simulink model "SF103A_MotRefMdl"  (R2013b)
settings: Solver=FixedStepDiscrete  StartTime=0.0  StopTime=2  FixedStep=.002  RelTol=1e-3
values from neighbouring files (symbols this model uses):
  ARCHGLBPRM_2MILLISEC_SEC_F32 = DataDict.Constant    [SF103A_MotRefMdl_DataDict.m]
  ARCHGLBPRM_2OVERSQRT3_ULS_F32 = DataDict.Constant    [SF103A_MotRefMdl_DataDict.m]
  ARCHGLBPRM_2PI_ULS_F32 = DataDict.Constant    [SF103A_MotRefMdl_DataDict.m]
  ARCHGLBPRM_4OVERSQRT3_ULS_F32 = DataDict.Constant    [SF103A_MotRefMdl_DataDict.m]
  ARCHGLBPRM_5PIOVER4_ULS_F32 = DataDict.Constant    [SF103A_MotRefMdl_DataDict.m]
  ARCHGLBPRM_FLOATZEROTHD_ULS_F32 = DataDict.Constant    [SF103A_MotRefMdl_DataDict.m]
  ARCHGLBPRM_HALFSQRT3_ULS_F32 = DataDict.Constant    [SF103A_MotRefMdl_DataDict.m]
  ARCHGLBPRM_PI_ULS_F32 = DataDict.Constant    [SF103A_MotRefMdl_DataDict.m]
  MotRefMdlCurrDaxBoostGain = DataDict.Calibration    [SF103A_MotRefMdl_DataDict.m]
  MotRefMdlCurrDaxQaxRefDelta = DataDict.Calibration    [SF103A_MotRefMdl_DataDict.m]
  MotRefMdlCurrItrnTolr = DataDict.Calibration    [SF103A_MotRefMdl_DataDict.m]
  MotRefMdlFbCtrlDi = DataDict.Calibration    [SF103A_MotRefMdl_DataDict.m]
  MotRefMdlIvtrDeadTiBrdgVltgSca = DataDict.Calibration    [SF103A_MotRefMdl_DataDict.m]
  MotRefMdlMinCurrItrnLim = DataDict.Calibration    [SF103A_MotRefMdl_DataDict.m]
  MotRefMdlMotCurrDaxMaxSca = DataDict.Calibration    [SF103A_MotRefMdl_DataDict.m]
  MotRefMdlMotVltgDerivtvTiCon = DataDict.Calibration    [SF103A_MotRefMdl_DataDict.m]
  MotRefMdlRefLocnItrnLim = DataDict.Calibration    [SF103A_MotRefMdl_DataDict.m]
  MotRefMdlTqItrnLim = DataDict.Calibration    [SF103A_MotRefMdl_DataDict.m]
  MotRefMdlTqItrnTolr = DataDict.Calibration    [SF103A_MotRefMdl_DataDict.m]
  MotRefMdlVltgModDynCmpEna = DataDict.Calibration    [SF103A_MotRefMdl_DataDict.m]
  MotRefMdlVltgOverRThdSca = DataDict.Calibration    [SF103A_MotRefMdl_DataDict.m]
  SysGlbPrmMotPoleCnt = DataDict.ImprtdCal    [SF103A_MotRefMdl_DataDict.m]
undefined symbols (not defined in the file or in its folder): MotQuad1
libraries: NxtrLim x18, simulink x4, LnrIntrpn x3, Fil x2, NxtrAbslt x2, FixdToFloat x2, FloatToFixd x2, NxtrMath x1
(part 5 of 7)

== system SF103A_MotRefMdl/MotRefMdl/MotRefMdlPer1/LocateRef/F_VoltTest_2 ==
  note: Logic in model matches EA3 code implementation.
      | Equivalent logic to requirements.  IF A >=B THEN true, vs. IF A<B THEN false
  VdR_Amp : Inport  RequirementInfo={} %GIDa_bdbdc2c3_337f_4636_8500_24b9b9be1375
  VqR_Amp : Inport  RequirementInfo={} %GIDa_c695ae3b_f6f3_41a1_91ce_9f5336ca82de  Port=2
  IntermediateCalcs : Inport  RequirementInfo={} %GIDa_c219b66e_6833_46f7_a9a0_194feb2a2a85  Port=3
  Add : Sum  RequirementInfo="{'linktype_rmi_doors' '0000bb42 (/E-STEER Core/SubSystem Specifications/Application Functions/SF99/SF103A Motor Reference Model)' '#SF103A_119' 'true' 'REQ:  SF103A_119' '' } %GIDa_dbf107c3_9fa7_4009_a0be_b6e3fb344bda"
  Bus Selector1 : BusSelector  RequirementInfo={} %GIDa_33d2b723_e6df_4a33_8d40_d160954a0577  OutputSignals=VovrRAllSqd_AmprSqd
  CopyRight2 : Subsystem  Description=|  mask(Copyright Information){none=on}
      | Copyright info block.                                               
      |                                                                     
      | Place copyright information at the top of every subsystem in design.
      mask prompts: none "No parameters"
      mask help: Place copyright information at the top of every subsystem in design.
      mask Display:
      | NxtrConf = 'Nexteer Confidential';
      | 
      | sys = bdroot; %handle for the current model ("system")
      | first = get_param(sys,'Created');
      | first = first(end-3:end);  %year is last four digits
      | 
      | last = get_param(sys,'LastModifiedDate');
      | if isempty(last)
      |     last = datestr(now,'yyyy');
      | else
      |     last = last(end-3:end);
      | end
      | 
      | if strcmp(first,last)
      |     fprintf('%s -- Copyright %s Nexteer',NxtrConf,first)
      | else
      |     fprintf('%s -- %s%s- %s Nexteer',NxtrConf,char(169),first,last)
      | end
  FALSE : Constant  RequirementInfo="{'linktype_rmi_doors' '0000bb42 (/E-STEER Core/SubSystem Specifications/Application Functions/SF99/SF103A Motor Reference Model)' '#SF103A_119' 'true' 'REQ:  SF103A_119' '' } %GIDa_ee86af96_5ed4_44a6_8699_a19f428d2a54"  Value=false  OutDataTypeStr=boolean
  FALSE1 : Constant  RequirementInfo="{'linktype_rmi_doors' '0000bb42 (/E-STEER Core/SubSystem Specifications/Application Functions/SF99/SF103A Motor Reference Model)' '#SF103A_119' 'true' 'REQ:  SF103A_119' '' } %GIDa_1262f9f4_0d67_49d1_9a04_2ae3e320c696"  Value=true  OutDataTypeStr=boolean
  If : If  RequirementInfo="{'linktype_rmi_doors' '0000bb42 (/E-STEER Core/SubSystem Specifications/Application Functions/SF99/SF103A Motor Reference Model)' '#SF103A_119' 'true' 'REQ:  SF103A_119' '' } %GIDa_d42d34e1_4d2b_4151_9a85_4eaef8bbfccb"  NumInputs=2  IfExpression=u1 < u2
  Math Function : Math  RequirementInfo="{'linktype_rmi_doors' '0000bb42 (/E-STEER Core/SubSystem Specifications/Application Functions/SF99/SF103A Motor Reference Model)' '#SF103A_119' 'true' 'REQ:  SF103A_119' '' } %GIDa_8409f596_67f9_422a_ad58_842fda6fb30d"  Operator=square  SaturateOnIntegerOverflow=on
  Math Function1 : Math  RequirementInfo="{'linktype_rmi_doors' '0000bb42 (/E-STEER Core/SubSystem Specifications/Application Functions/SF99/SF103A Motor Reference Model)' '#SF103A_119' 'true' 'REQ:  SF103A_119' '' } %GIDa_805105ee_f5aa_4ac0_bbbc_edf23613534f"  Operator=square  SaturateOnIntegerOverflow=on
  Merge : Merge  RequirementInfo="{'linktype_rmi_doors' '0000bb42 (/E-STEER Core/SubSystem Specifications/Application Functions/SF99/SF103A Motor Reference Model)' '#SF103A_119' 'true' 'REQ:  SF103A_119' '' } %GIDa_7c079081_5a0f_4465_b1a6_f75de5ead0d0"
  set_false : Subsystem  RequirementInfo="{'linktype_rmi_doors' '0000bb42 (/E-STEER Core/SubSystem Specifications/Application Functions/SF99/SF103A Motor Reference Model)' '#SF103A_119' 'true' 'REQ:  SF103A_119' '' } %GIDa_10e3cc76_5863_44c3_b625_9632a7c78e0a"  TreatAsAtomicUnit=on
  set_true : Subsystem  RequirementInfo="{'linktype_rmi_doors' '0000bb42 (/E-STEER Core/SubSystem Specifications/Application Functions/SF99/SF103A Motor Reference Model)' '#SF103A_119' 'true' 'REQ:  SF103A_119' '' } %GIDa_040fa8b4_6b1a_42f0_bcc2_e676a9d0bb48"  TreatAsAtomicUnit=on
  VoltTest_Uls : Outport  RequirementInfo={} %GIDa_3e99ad84_82c1_4399_8e9b_f18249aabee0
  wires:
  IntermediateCalcs/1 -> Bus Selector1/1
  Bus Selector1/1 -> If/2  "<VovrRAllSqd_AmprSqd>"
  VdR_Amp/1 -> Math Function/1  "VdR_Amp"
  VqR_Amp/1 -> Math Function1/1  "VqR_Amp"
  Math Function/1 -> Add/1
  Math Function1/1 -> Add/2
  Add/1 -> If/1  "Vdq_AmpSq_T_f32"
  If/1 -> set_false/Action
  If/2 -> set_true/Action
  FALSE/1 -> set_false/1(In1)
  FALSE1/1 -> set_true/1(In1)
  set_false/1(Out1) -> Merge/1
  set_true/1(Out1) -> Merge/2
  Merge/1 -> VoltTest_Uls/1

== system SF103A_MotRefMdl/MotRefMdl/MotRefMdlPer1/LocateRef/for_loop_stuff_here ==
  InterCalcns : Inport
  IdMax_Amp : Inport  Port=2
  IdMin_Amp : Inport  Port=3
  MotTqCmd : Inport  Port=4
  Action Port : ActionPort  ActionType=else
  Constant1 : Constant  Value=MotRefMdlRefLocnItrnLim
  CopyRight2 : Subsystem  Description=|  mask(Copyright Information){none=on}
      | Copyright info block.                                               
      |                                                                     
      | Place copyright information at the top of every subsystem in design.
      mask prompts: none "No parameters"
      mask help: Place copyright information at the top of every subsystem in design.
      mask Display:
      | NxtrConf = 'Nexteer Confidential';
      | 
      | sys = bdroot; %handle for the current model ("system")
      | first = get_param(sys,'Created');
      | first = first(end-3:end);  %year is last four digits
      | 
      | last = get_param(sys,'LastModifiedDate');
      | if isempty(last)
      |     last = datestr(now,'yyyy');
      | else
      |     last = last(end-3:end);
      | end
      | 
      | if strcmp(first,last)
      |     fprintf('%s -- Copyright %s Nexteer',NxtrConf,first)
      | else
      |     fprintf('%s -- %s%s- %s Nexteer',NxtrConf,char(169),first,last)
      | end
  For Iterator Subsystem : Subsystem  TreatAsAtomicUnit=on
  Mux1 : Mux
  Refs : Outport
  wires:
  InterCalcns/1 -> For Iterator Subsystem/4(InterCalcns)
  For Iterator Subsystem/1(IdMid_Amp) -> Mux1/1
  For Iterator Subsystem/2(IqMid_Amp) -> Mux1/2
  IdMax_Amp/1 -> For Iterator Subsystem/1(IdMax_Amp)
  IdMin_Amp/1 -> For Iterator Subsystem/2(IdMin_Amp)
  MotTqCmd/1 -> For Iterator Subsystem/3(MotTqCmd)
  Constant1/1 -> For Iterator Subsystem/5(IterLim)
  For Iterator Subsystem/3(VdR) -> Mux1/3
  For Iterator Subsystem/4(VqR) -> Mux1/4
  Mux1/1 -> Refs/1

== system SF103A_MotRefMdl/MotRefMdl/MotRefMdlPer1/LocateRef/pass_thru_1 ==
  in1 : Inport
  Action Port : ActionPort  ActionType=then
  out1 : Outport
  wires:
  in1/1 -> out1/1

== system SF103A_MotRefMdl/MotRefMdl/MotRefMdlPer1/LocateRef/pass_thru_2 ==
  in1 : Inport
  Action Port : ActionPort  ActionType=elseif
  out1 : Outport
  wires:
  in1/1 -> out1/1

== system SF103A_MotRefMdl/MotRefMdl/MotRefMdlPer1/LocateTorqueExtremes/CalculateTorque ==
  CurrDax : Inport  RequirementInfo={} %GIDa_2998f73f_9d72_4bd2_aa74_a01c2b485170
  CurrQax : Inport  RequirementInfo={} %GIDa_ca6dbf11_0384_4fff_ba84_da57f1286247  Port=2
  In2 : Inport  RequirementInfo={} %GIDa_4eca7850_e42c_48c4_b2e6_d9b51f8c8086  Port=3
  Add1 : Sum  RequirementInfo="{'linktype_rmi_doors' '0000bb42 (/E-STEER Core/SubSystem Specifications/Application Functions/SF99/SF103A Motor Reference Model)' '#SF103A_95' 'true' 'REQ:  SF103A_95' '' } %GIDa_35104bf2_433c_40bb_9a03_9bef4e2662a2"
  Bus Selector2 : BusSelector  RequirementInfo={} %GIDa_2406d6d2_4952_432f_b9c9_4ab0e99a532f  OutputSignals=RelncTqCoeff_Henry_f32,Ke_VoltPerRadPerSec
  CopyRight2 : Subsystem  Description=|  mask(Copyright Information){none=on}
      | Copyright info block.                                               
      |                                                                     
      | Place copyright information at the top of every subsystem in design.
      mask prompts: none "No parameters"
      mask help: Place copyright information at the top of every subsystem in design.
      mask Display:
      | NxtrConf = 'Nexteer Confidential';
      | 
      | sys = bdroot; %handle for the current model ("system")
      | first = get_param(sys,'Created');
      | first = first(end-3:end);  %year is last four digits
      | 
      | last = get_param(sys,'LastModifiedDate');
      | if isempty(last)
      |     last = datestr(now,'yyyy');
      | else
      |     last = last(end-3:end);
      | end
      | 
      | if strcmp(first,last)
      |     fprintf('%s -- Copyright %s Nexteer',NxtrConf,first)
      | else
      |     fprintf('%s -- %s%s- %s Nexteer',NxtrConf,char(169),first,last)
      | end
  Product4 : Product  RequirementInfo="{'linktype_rmi_doors' '0000bb42 (/E-STEER Core/SubSystem Specifications/Application Functions/SF99/SF103A Motor Reference Model)' '#SF103A_95' 'true' 'REQ:  SF103A_95' '' } %GIDa_6ad1e118_1952_4c77_ba9a_8385ef3a4332"
  Product5 : Product  RequirementInfo="{'linktype_rmi_doors' '0000bb42 (/E-STEER Core/SubSystem Specifications/Application Functions/SF99/SF103A Motor Reference Model)' '#SF103A_95' 'true' 'REQ:  SF103A_95' '' } %GIDa_2fded1a9_a815_47ff_97c2_8d512119d41f"
  TqAry : Outport  RequirementInfo={} %GIDa_95062886_6bc0_4d5b_80ab_b3af293c4ad7
  wires:
  CurrDax/1 -> Product4/1
  Bus Selector2/1 -> Product4/2  "<RelncTqCoeff_Henry_f32>"
  Bus Selector2/2 -> Add1/2  "<Ke_VoltPerRadPerSec>"
  Product4/1 -> Add1/1
  Add1/1 -> Product5/2
  Product5/1 -> TqAry/1  "TqAry"
  CurrQax/1 -> Product5/1
  In2/1 -> Bus Selector2/1

== system SF103A_MotRefMdl/MotRefMdl/MotRefMdlPer1/LocateTorqueExtremes/CopyRight2 ==

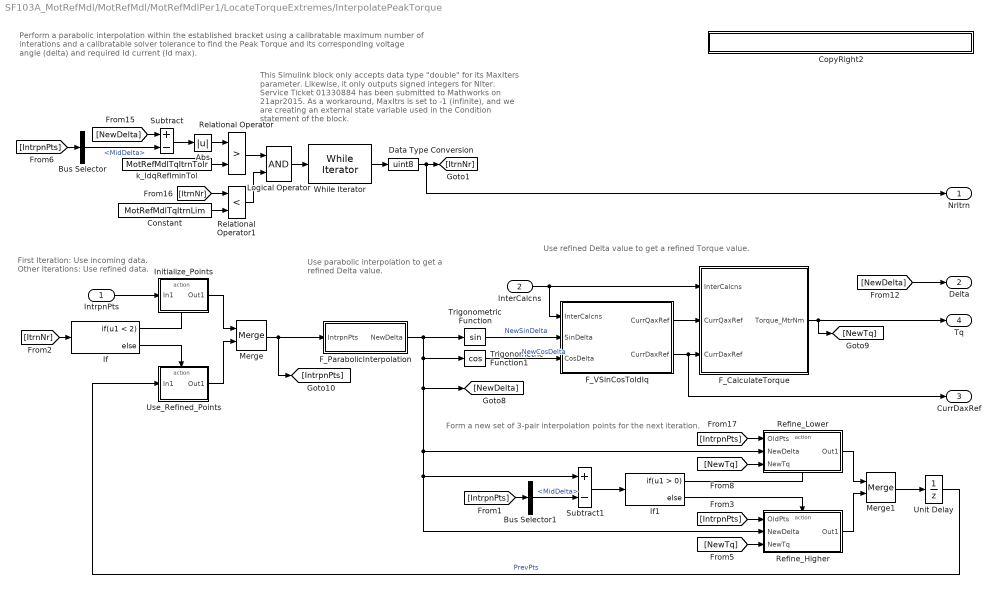
== system SF103A_MotRefMdl/MotRefMdl/MotRefMdlPer1/LocateTorqueExtremes/InterpolatePeakTorque ==
  note: Perform a parabolic interpolation within the established bracket using a calibratable maximum number of interations and
      | a calibratable solver tolerance to find the Peak Torque and its corresponding voltage angle (delta) and required Id current (Id max).
  note: Form a new set of 3-pair interpolation points for the next iteration.
  note: Use refined Delta value to get a refined Torque value.
  note: Use parabolic interpolation to get
      | a refined Delta value.
  note: First Iteration:      Use incoming data.
      | Other Iterations:  Use refined data.
  note: This Simulink block only accepts data type "double" for its MaxIters parameter.
      | Likewise, it only outputs signed integers for NIter.
      | Service Ticket 01330884 has been submitted to Mathworks on 21apr2015.
      |
      | As a workaround, MaxItrs is set to -1 (infinite), and we are creating an external
      | state variable used in the Condition statement of the block.
  IntrpnPts : Inport  RequirementInfo={} %GIDa_2976d57d_e282_4f49_8a63_56b19d06b85b
  InterCalcns : Inport  RequirementInfo={} %GIDa_a716d5ab_e582_42aa_b641_9b315bdd793f  Port=2
  Abs : Abs  RequirementInfo="{'linktype_rmi_doors' '0000bb42 (/E-STEER Core/SubSystem Specifications/Application Functions/SF99/SF103A Motor Reference Model)' '#SF103A_138' 'true' 'REQ:  SF103A_138' '' } %GIDa_dbcfb43a_3396_4992_a45f_a8a74d44d3a7"
  Bus Selector : BusSelector  RequirementInfo={} %GIDa_7e8a8e4b_2db3_43c1_ad91_ebf4492f1ebf  OutputSignals=MidDelta
  Bus Selector1 : BusSelector  RequirementInfo={} %GIDa_e4020d49_c2af_4ccf_99e4_5a477bc0dbad  OutputSignals=MidDelta
  Constant : Constant  RequirementInfo="{'linktype_rmi_doors' '0000bb42 (/E-STEER Core/SubSystem Specifications/Application Functions/SF99/SF103A Motor Reference Model)' '#SF103A_138' 'true' 'REQ:  SF103A_138' '' } %GIDa_9a6db34d_4491_4dbd_827c_4bf42d84f720"  Value=MotRefMdlTqItrnLim
  CopyRight2 : Subsystem  Description=|  mask(Copyright Information){none=on}
      | Copyright info block.                                               
      |                                                                     
      | Place copyright information at the top of every subsystem in design.
      mask prompts: none "No parameters"
      mask help: Place copyright information at the top of every subsystem in design.
      mask Display:
      | NxtrConf = 'Nexteer Confidential';
      | 
      | sys = bdroot; %handle for the current model ("system")
      | first = get_param(sys,'Created');
      | first = first(end-3:end);  %year is last four digits
      | 
      | last = get_param(sys,'LastModifiedDate');
      | if isempty(last)
      |     last = datestr(now,'yyyy');
      | else
      |     last = last(end-3:end);
      | end
      | 
      | if strcmp(first,last)
      |     fprintf('%s -- Copyright %s Nexteer',NxtrConf,first)
      | else
      |     fprintf('%s -- %s%s- %s Nexteer',NxtrConf,char(169),first,last)
      | end
  Data Type Conversion : DataTypeConversion  RequirementInfo="{'linktype_rmi_doors' '0000bb42 (/E-STEER Core/SubSystem Specifications/Application Functions/SF99/SF103A Motor Reference Model)' '#SF103A_138' 'true' 'REQ:  SF103A_138' '' } %GIDa_d05ab658_2675_4616_9556_eb4a3e433000"  OutDataTypeStr=uint8
  F_CalculateTorque : Subsystem  RequirementInfo="{'linktype_rmi_doors' '0000bb42 (/E-STEER Core/SubSystem Specifications/Application Functions/SF99/SF103A Motor Reference Model)' '#SF103A_138' 'true' 'REQ:  SF103A_138' '' } %GIDa_fb42ee02_0f3e_4705_9759_bd25b532bd66"
  F_ParabolicInterpolation : Subsystem  RequirementInfo="{'linktype_rmi_doors' '0000bb42 (/E-STEER Core/SubSystem Specifications/Application Functions/SF99/SF103A Motor Reference Model)' '#SF103A_101' 'true' 'REQ:  SF103A_101' '' } %GIDa_0053af21_204c_49c7_9cc1_22fea14c8add"
  F_VSinCosToIdIq : Subsystem  RequirementInfo="{'linktype_rmi_doors' '0000bb42 (/E-STEER Core/SubSystem Specifications/Application Functions/SF99/SF103A Motor Reference Model)' '#SF103A_138' 'true' 'REQ:  SF103A_138' '' } %GIDa_7cfa491a_5909_4b64_979d_2d83487ab5dd"
  If : If  RequirementInfo="{'linktype_rmi_doors' '0000bb42 (/E-STEER Core/SubSystem Specifications/Application Functions/SF99/SF103A Motor Reference Model)' '#SF103A_138' 'true' 'REQ:  SF103A_138' '' } %GIDa_99f7b3ff_37c2_4b5c_b2d2_7b22340d00ca"  IfExpression=u1 < 2
  If1 : If  RequirementInfo="{'linktype_rmi_doors' '0000bb42 (/E-STEER Core/SubSystem Specifications/Application Functions/SF99/SF103A Motor Reference Model)' '#SF103A_138' 'true' 'REQ:  SF103A_138' '' } %GIDa_8d1be50d_692b_4f8b_8365_dcaa30d6a252"
  Initialize_Points : Subsystem  RequirementInfo="{'linktype_rmi_doors' '0000bb42 (/E-STEER Core/SubSystem Specifications/Application Functions/SF99/SF103A Motor Reference Model)' '#SF103A_138' 'true' 'REQ:  SF103A_138' '' } %GIDa_bec8c2c2_f944_41e2_9ca7_df93196ca809"  TreatAsAtomicUnit=on
  Logical Operator : Logic  RequirementInfo="{'linktype_rmi_doors' '0000bb42 (/E-STEER Core/SubSystem Specifications/Application Functions/SF99/SF103A Motor Reference Model)' '#SF103A_138' 'true' 'REQ:  SF103A_138' '' } %GIDa_6ff35568_919a_4eb8_adae_75a9800725bf"  AllPortsSameDT=off  OutDataTypeStr=boolean
  Merge : Merge  RequirementInfo="{'linktype_rmi_doors' '0000bb42 (/E-STEER Core/SubSystem Specifications/Application Functions/SF99/SF103A Motor Reference Model)' '#SF103A_138' 'true' 'REQ:  SF103A_138' '' } %GIDa_0e8b307d_47aa_40fc_9a54_6513a36a9b6b"
  Merge1 : Merge  RequirementInfo="{'linktype_rmi_doors' '0000bb42 (/E-STEER Core/SubSystem Specifications/Application Functions/SF99/SF103A Motor Reference Model)' '#SF103A_138' 'true' 'REQ:  SF103A_138' '' } %GIDa_04bf0c78_d0d1_43d8_90f1_17c925cfd637"
  Refine_Higher : Subsystem  RequirementInfo="{'linktype_rmi_doors' '0000bb42 (/E-STEER Core/SubSystem Specifications/Application Functions/SF99/SF103A Motor Reference Model)' '#SF103A_138' 'true' 'REQ:  SF103A_138' '' } %GIDa_f9b8b134_eccc_466f_ba96_ac0bcc73a754"  TreatAsAtomicUnit=on
  Refine_Lower : Subsystem  RequirementInfo="{'linktype_rmi_doors' '0000bb42 (/E-STEER Core/SubSystem Specifications/Application Functions/SF99/SF103A Motor Reference Model)' '#SF103A_138' 'true' 'REQ:  SF103A_138' '' } %GIDa_2bb29e56_5ec3_4499_9866_34e197e89fba"  TreatAsAtomicUnit=on
  Relational Operator : RelationalOperator  RequirementInfo="{'linktype_rmi_doors' '0000bb42 (/E-STEER Core/SubSystem Specifications/Application Functions/SF99/SF103A Motor Reference Model)' '#SF103A_138' 'true' 'REQ:  SF103A_138' '' } %GIDa_66b7cfce_1756_4987_b74a_12ef9cfeba9f"  Operator=>  OutDataTypeStr=boolean
  Relational Operator1 : RelationalOperator  RequirementInfo="{'linktype_rmi_doors' '0000bb42 (/E-STEER Core/SubSystem Specifications/Application Functions/SF99/SF103A Motor Reference Model)' '#SF103A_138' 'true' 'REQ:  SF103A_138' '' } %GIDa_5ddb5cd4_2348_4b9d_a919_db26decc9c0e"  Operator=<  OutDataTypeStr=boolean
  Subtract : Sum  RequirementInfo="{'linktype_rmi_doors' '0000bb42 (/E-STEER Core/SubSystem Specifications/Application Functions/SF99/SF103A Motor Reference Model)' '#SF103A_138' 'true' 'REQ:  SF103A_138' '' } %GIDa_bf0c4dbf_6147_44dd_82af_70477d657d08"  Inputs=+-
  Subtract1 : Sum  RequirementInfo="{'linktype_rmi_doors' '0000bb42 (/E-STEER Core/SubSystem Specifications/Application Functions/SF99/SF103A Motor Reference Model)' '#SF103A_138' 'true' 'REQ:  SF103A_138' '' } %GIDa_1494702e_ee4e_4592_b03b_ab6118063e27"  Inputs=+-
  Trigonometric Function : Trigonometry  RequirementInfo="{'linktype_rmi_doors' '0000bb42 (/E-STEER Core/SubSystem Specifications/Application Functions/SF99/SF103A Motor Reference Model)' '#SF103A_138' 'true' 'REQ:  SF103A_138' '' } %GIDa_16ec79dd_c639_471c_bd6c_7a1cc3dcc806"
  Trigonometric Function1 : Trigonometry  RequirementInfo="{'linktype_rmi_doors' '0000bb42 (/E-STEER Core/SubSystem Specifications/Application Functions/SF99/SF103A Motor Reference Model)' '#SF103A_138' 'true' 'REQ:  SF103A_138' '' } %GIDa_81905544_8884_4996_930f_48fbf37d91af"  Operator=cos
  Unit Delay : UnitDelay  RequirementInfo="{'linktype_rmi_doors' '0000bb42 (/E-STEER Core/SubSystem Specifications/Application Functions/SF99/SF103A Motor Reference Model)' '#SF103A_138' 'true' 'REQ:  SF103A_138' '' } %GIDa_a28fdb37_551d_4b3e_85eb_2b6c47a2de6c"  SampleTime=-1
      settings: AttributesFormatString=|
      | Temp Variable
      | No PIM
  Use_Refined_Points : Subsystem  RequirementInfo="{'linktype_rmi_doors' '0000bb42 (/E-STEER Core/SubSystem Specifications/Application Functions/SF99/SF103A Motor Reference Model)' '#SF103A_138' 'true' 'REQ:  SF103A_138' '' } %GIDa_4ca1c458_5610_48fc_b3a4_dad5a3a0bbe1"  TreatAsAtomicUnit=on
  While Iterator : WhileIterator  RequirementInfo="{'linktype_rmi_doors' '0000bb42 (/E-STEER Core/SubSystem Specifications/Application Functions/SF99/SF103A Motor Reference Model)' '#SF103A_138' 'true' 'REQ:  SF103A_138' '' } %GIDa_0c316dfc_7e56_439b_9700_2def35b71c1c"  MaxIters=-1  WhileBlockType=do-while  ShowIterationPort=on  OutputDataType=int8
      settings: AttributesFormatString=%<MaxIters>
  k_IdqRefIminTol : Constant  RequirementInfo="{'linktype_rmi_doors' '0000bb42 (/E-STEER Core/SubSystem Specifications/Application Functions/SF99/SF103A Motor Reference Model)' '#SF103A_138' 'true' 'REQ:  SF103A_138' '' } %GIDa_82618eb1_9771_4ab5_ad22_c97f24fa1b2b"  Value=MotRefMdlTqItrnTolr
  NrItrn : Outport  RequirementInfo={} %GIDa_a221836d_0b58_44bc_ab39_f81c5b30c4c7
  Delta : Outport  RequirementInfo={} %GIDa_1f963225_897f_46a2_9740_bc657ff62af4  Port=2
  CurrDaxRef : Outport  RequirementInfo={} %GIDa_1c11b45b_d613_4d33_bfb8_c16146ea4818  Port=3
  Tq : Outport  RequirementInfo={} %GIDa_902077c8_9265_4b3a_8b2e_6b417a4e4d03  Port=4
  wires:
  F_CalculateTorque/1(Torque_MtrNm) -> [NewTq], Tq/1
  InterCalcns/1 -> F_VSinCosToIdIq/1(InterCalcns), F_CalculateTorque/1(InterCalcns)
  While Iterator/1 -> Data Type Conversion/1
  Merge1/1 -> Unit Delay/1
  Subtract/1 -> Abs/1
  Relational Operator/1 -> Logical Operator/1
  [NewDelta] -> Subtract/1
  [ItrnNr] -> Relational Operator1/1
  Constant/1 -> Relational Operator1/2
  Logical Operator/1 -> While Iterator/1
  Relational Operator1/1 -> Logical Operator/2
  [IntrpnPts] -> Bus Selector/1
  Bus Selector/1 -> Subtract/2  "<MidDelta>"
  IntrpnPts/1 -> Initialize_Points/1(In1)
  [ItrnNr] -> If/1
  Unit Delay/1 -> Use_Refined_Points/1(In1)  "PrevPts"
  If1/1 -> Refine_Lower/Action
  If1/2 -> Refine_Higher/Action
  Refine_Lower/1(Out1) -> Merge1/1
  Refine_Higher/1(Out1) -> Merge1/2
  [IntrpnPts] -> Refine_Lower/1(OldPts)
  [IntrpnPts] -> Refine_Higher/1(OldPts)
  [NewTq] -> Refine_Lower/3(NewTq)
  Merge/1 -> [IntrpnPts], F_ParabolicInterpolation/1(IntrpnPts)
  [IntrpnPts] -> Bus Selector1/1
  Bus Selector1/1 -> Subtract1/2  "<MidDelta>"
  Subtract1/1 -> If1/1
  F_ParabolicInterpolation/1(NewDelta) -> Trigonometric Function/1, [NewDelta], Refine_Lower/2(NewDelta), Refine_Higher/2(NewDelta), Subtract1/1, Trigonometric Function1/1
  [NewTq] -> Refine_Higher/3(NewTq)
  If/1 -> Initialize_Points/Action
  If/2 -> Use_Refined_Points/Action
  Initialize_Points/1(Out1) -> Merge/1
  Use_Refined_Points/1(Out1) -> Merge/2
  Data Type Conversion/1 -> NrItrn/1, [ItrnNr]
  Abs/1 -> Relational Operator/1
  k_IdqRefIminTol/1 -> Relational Operator/2
  [NewDelta] -> Delta/1
  Trigonometric Function/1 -> F_VSinCosToIdIq/2(SinDelta)  "NewSinDelta"
  Trigonometric Function1/1 -> F_VSinCosToIdIq/3(CosDelta)  "NewCosDelta"
  F_VSinCosToIdIq/2(CurrDaxRef) -> CurrDaxRef/1, F_CalculateTorque/3(CurrDaxRef)
  F_VSinCosToIdIq/1(CurrQaxRef) -> F_CalculateTorque/2(CurrQaxRef)

== system SF103A_MotRefMdl/MotRefMdl/MotRefMdlPer1/LocateTorqueExtremes/Negative ==
  TqAry : Inport
  Action Port : ActionPort  ActionType=else
  CopyRight2 : Subsystem  Description=|  mask(Copyright Information){none=on}
      | Copyright info block.                                               
      |                                                                     
      | Place copyright information at the top of every subsystem in design.
      mask prompts: none "No parameters"
      mask help: Place copyright information at the top of every subsystem in design.
      mask Display:
      | NxtrConf = 'Nexteer Confidential';
      | 
      | sys = bdroot; %handle for the current model ("system")
      | first = get_param(sys,'Created');
      | first = first(end-3:end);  %year is last four digits
      | 
      | last = get_param(sys,'LastModifiedDate');
      | if isempty(last)
      |     last = datestr(now,'yyyy');
      | else
      |     last = last(end-3:end);
      | end
      | 
      | if strcmp(first,last)
      |     fprintf('%s -- Copyright %s Nexteer',NxtrConf,first)
      | else
      |     fprintf('%s -- %s%s- %s Nexteer',NxtrConf,char(169),first,last)
      | end
  For Iterator Subsystem : Subsystem  TreatAsAtomicUnit=on
  IdxSt : Outport
  wires:
  TqAry/1 -> For Iterator Subsystem/1(TqAry)
  For Iterator Subsystem/1(IdxSt) -> IdxSt/1

== system SF103A_MotRefMdl/MotRefMdl/MotRefMdlPer1/LocateTorqueExtremes/Positive ==
  TqAry : Inport
  Action Port : ActionPort  ActionType=then
  CopyRight2 : Subsystem  Description=|  mask(Copyright Information){none=on}
      | Copyright info block.                                               
      |                                                                     
      | Place copyright information at the top of every subsystem in design.
      mask prompts: none "No parameters"
      mask help: Place copyright information at the top of every subsystem in design.
      mask Display:
      | NxtrConf = 'Nexteer Confidential';
      | 
      | sys = bdroot; %handle for the current model ("system")
      | first = get_param(sys,'Created');
      | first = first(end-3:end);  %year is last four digits
      | 
      | last = get_param(sys,'LastModifiedDate');
      | if isempty(last)
      |     last = datestr(now,'yyyy');
      | else
      |     last = last(end-3:end);
      | end
      | 
      | if strcmp(first,last)
      |     fprintf('%s -- Copyright %s Nexteer',NxtrConf,first)
      | else
      |     fprintf('%s -- %s%s- %s Nexteer',NxtrConf,char(169),first,last)
      | end
  For Iterator Subsystem : Subsystem  TreatAsAtomicUnit=on
  IdxSt : Outport
  wires:
  TqAry/1 -> For Iterator Subsystem/1(TqAry)
  For Iterator Subsystem/1(IdxSt) -> IdxSt/1

== system SF103A_MotRefMdl/MotRefMdl/MotRefMdlPer1/LocateTorqueExtremes/WrapBracketAngles ==
  note: Creates a bracket around the peak torque from the Find Peak Torque step, in order to set up a finer search
      | to find a more accurate peak torque.  To ensure there are no errors in interpolation, if the peak torque is at
      | an end point of the array, the angles are "wrapped".
  note: NOTE: Zero-based indexing
  TqAry : Inport  RequirementInfo={} %GIDa_236e65cd_bd1d_4674_bd97_cda757c01c81
  IdxSt : Inport  RequirementInfo={} %GIDa_6c627307_0a2d_4e0a_9d77_e9d62fef5486  Port=2
  CopyRight2 : Subsystem  Description=|  mask(Copyright Information){none=on}
      | Copyright info block.                                               
      |                                                                     
      | Place copyright information at the top of every subsystem in design.
      mask prompts: none "No parameters"
      mask help: Place copyright information at the top of every subsystem in design.
      mask Display:
      | NxtrConf = 'Nexteer Confidential';
      | 
      | sys = bdroot; %handle for the current model ("system")
      | first = get_param(sys,'Created');
      | first = first(end-3:end);  %year is last four digits
      | 
      | last = get_param(sys,'LastModifiedDate');
      | if isempty(last)
      |     last = datestr(now,'yyyy');
      | else
      |     last = last(end-3:end);
      | end
      | 
      | if strcmp(first,last)
      |     fprintf('%s -- Copyright %s Nexteer',NxtrConf,first)
      | else
      |     fprintf('%s -- %s%s- %s Nexteer',NxtrConf,char(169),first,last)
      | end
  If : If  RequirementInfo="{'linktype_rmi_doors' '0000bb42 (/E-STEER Core/SubSystem Specifications/Application Functions/SF99/SF103A Motor Reference Model)' '#SF103A_138' 'true' 'REQ:  SF103A_138' '' ; 'linktype_rmi_doors' '0000bb42 (/E-STEER Core/SubSystem Specifications/Application Functions/SF99/SF103A Motor Reference Model)' '#SF103A_100' 'true' 'REQ:  SF103A_100' '' } %GIDa_534a1ceb_7e41_4741_9b68_810f1f2c2b7b"  IfExpression=u1 == 0  ElseIfExpressions=u1 == 7
  Merge : Merge  RequirementInfo="{'linktype_rmi_doors' '0000bb42 (/E-STEER Core/SubSystem Specifications/Application Functions/SF99/SF103A Motor Reference Model)' '#SF103A_138' 'true' 'REQ:  SF103A_138' '' ; 'linktype_rmi_doors' '0000bb42 (/E-STEER Core/SubSystem Specifications/Application Functions/SF99/SF103A Motor Reference Model)' '#SF103A_100' 'true' 'REQ:  SF103A_100' '' } %GIDa_af647c15_115f_403d_af8f_beccccf209d9"  Inputs=3
  No_Wrapping : Subsystem  RequirementInfo="{'linktype_rmi_doors' '0000bb42 (/E-STEER Core/SubSystem Specifications/Application Functions/SF99/SF103A Motor Reference Model)' '#SF103A_138' 'true' 'REQ:  SF103A_138' '' ; 'linktype_rmi_doors' '0000bb42 (/E-STEER Core/SubSystem Specifications/Application Functions/SF99/SF103A Motor Reference Model)' '#SF103A_100' 'true' 'REQ:  SF103A_100' '' } %GIDa_b5248bab_61f6_4ee6_993a_50a1405399ed"  TreatAsAtomicUnit=on
      settings: RTWSystemCode=Inline
  Wrap_Lowr : Subsystem  RequirementInfo="{'linktype_rmi_doors' '0000bb42 (/E-STEER Core/SubSystem Specifications/Application Functions/SF99/SF103A Motor Reference Model)' '#SF103A_138' 'true' 'REQ:  SF103A_138' '' ; 'linktype_rmi_doors' '0000bb42 (/E-STEER Core/SubSystem Specifications/Application Functions/SF99/SF103A Motor Reference Model)' '#SF103A_100' 'true' 'REQ:  SF103A_100' '' } %GIDa_f29c4ee1_cfe5_4c87_9879_d6394633a975"  TreatAsAtomicUnit=on
      settings: RTWSystemCode=Inline
  Wrap_Uppr : Subsystem  RequirementInfo="{'linktype_rmi_doors' '0000bb42 (/E-STEER Core/SubSystem Specifications/Application Functions/SF99/SF103A Motor Reference Model)' '#SF103A_138' 'true' 'REQ:  SF103A_138' '' ; 'linktype_rmi_doors' '0000bb42 (/E-STEER Core/SubSystem Specifications/Application Functions/SF99/SF103A Motor Reference Model)' '#SF103A_100' 'true' 'REQ:  SF103A_100' '' } %GIDa_3a3eb958_cee3_46f8_90f2_778c7d1029b5"  TreatAsAtomicUnit=on
      settings: RTWSystemCode=Inline
  IntrpnPts : Outport  RequirementInfo={} %GIDa_bab3e613_be3c_449a_b074_a335cceeda09
  wires:
  Merge/1 -> IntrpnPts/1
  IdxSt/1 -> [index]
  TqAry/1 -> [torques]
  [index] -> If/1
  If/1 -> Wrap_Lowr/Action
  If/2 -> Wrap_Uppr/Action
  [index] -> Wrap_Lowr/2(Idx)
  If/3 -> No_Wrapping/Action
  Wrap_Lowr/1(IntrpnPts) -> Merge/1
  Wrap_Uppr/1(IntrpnPts) -> Merge/2
  No_Wrapping/1(IntrpnPts) -> Merge/3
  [torques] -> Wrap_Lowr/1(TqAry)
  [index] -> Wrap_Uppr/2(Idx)
  [torques] -> Wrap_Uppr/1(TqAry)
  [index] -> No_Wrapping/2(Idx)
  [torques] -> No_Wrapping/1(TqAry)

== system SF103A_MotRefMdl/MotRefMdl/MotRefMdlPer1/MotCurrAg_AlphaCalc/CopyRight2 ==

== system SF103A_MotRefMdl/MotRefMdl/MotRefMdlPer1/MotCurrAg_AlphaCalc/No Wrapping ==
  In1 : Inport
  Action Port : ActionPort  ActionType=else
  Out1 : Outport
  wires:
  In1/1 -> Out1/1

== system SF103A_MotRefMdl/MotRefMdl/MotRefMdlPer1/MotCurrAg_AlphaCalc/Wrap Angle ==
  In1 : Inport
  Action Port : ActionPort  ActionType=then
  Add : Sum
  Constant : Constant  Value=ARCHGLBPRM_2PI_ULS_F32
  CopyRight2 : Subsystem  Description=|  mask(Copyright Information){none=on}
      | Copyright info block.                                               
      |                                                                     
      | Place copyright information at the top of every subsystem in design.
      mask prompts: none "No parameters"
      mask help: Place copyright information at the top of every subsystem in design.
      mask Display:
      | NxtrConf = 'Nexteer Confidential';
      | 
      | sys = bdroot; %handle for the current model ("system")
      | first = get_param(sys,'Created');
      | first = first(end-3:end);  %year is last four digits
      | 
      | last = get_param(sys,'LastModifiedDate');
      | if isempty(last)
      |     last = datestr(now,'yyyy');
      | else
      |     last = last(end-3:end);
      | end
      | 
      | if strcmp(first,last)
      |     fprintf('%s -- Copyright %s Nexteer',NxtrConf,first)
      | else
      |     fprintf('%s -- %s%s- %s Nexteer',NxtrConf,char(169),first,last)
      | end
  Out1 : Outport
  wires:
  In1/1 -> Add/1
  Constant/1 -> Add/2
  Add/1 -> Out1/1

== system SF103A_MotRefMdl/MotRefMdl/MotRefMdlPer1/VoltageScheduling/CopyRight2 ==

== system SF103A_MotRefMdl/MotRefMdl/MotRefMdlPer1/VoltageScheduling/If Action Subsystem ==
  AbsMotVelFild : Inport  RequirementInfo={} %GIDa_3dd955b8_f6a9_429c_adbf_401cb09647a9
  Action Port : ActionPort  ActionType=then
  CopyRight2 : Subsystem  Description=|  mask(Copyright Information){none=on}
      | Copyright info block.                                               
      |                                                                     
      | Place copyright information at the top of every subsystem in design.
      mask prompts: none "No parameters"
      mask help: Place copyright information at the top of every subsystem in design.
      mask Display:
      | NxtrConf = 'Nexteer Confidential';
      | 
      | sys = bdroot; %handle for the current model ("system")
      | first = get_param(sys,'Created');
      | first = first(end-3:end);  %year is last four digits
      | 
      | last = get_param(sys,'LastModifiedDate');
      | if isempty(last)
      |     last = datestr(now,'yyyy');
      | else
      |     last = last(end-3:end);
      | end
      | 
      | if strcmp(first,last)
      |     fprintf('%s -- Copyright %s Nexteer',NxtrConf,first)
      | else
      |     fprintf('%s -- %s%s- %s Nexteer',NxtrConf,char(169),first,last)
      | end
  Quad_13_Budget : LnrIntrpn/LnrIntrpn_u16_u16VariXu16VariY  RequirementInfo="{'linktype_rmi_doors' '0000bb42 (/E-STEER Core/SubSystem Specifications/Application Functions/SF99/SF103A Motor Reference Model)' '#SF103A_75' 'true' 'REQ:  SF103A_75' '' } %GIDa_dc606676_1089_4e51_8278_f1eab2b8b263"  XTbl=MotRefMdlQuad13VltgSdlX  YTbl=MotRefMdlQuad13VltgSdlY
      settings: AttributesFormatString=Lnr ( u16VariX , u16VariY )
  VltgSdl : Outport  RequirementInfo={} %GIDa_3429f483_0239_4892_9589_5a88f57964d6
  wires:
  AbsMotVelFild/1 -> Quad_13_Budget/1
  Quad_13_Budget/1 -> VltgSdl/1

== system SF103A_MotRefMdl/MotRefMdl/MotRefMdlPer1/VoltageScheduling/If Action Subsystem1 ==
  AbsMotVelFild : Inport  RequirementInfo={} %GIDa_ff250ae2_f170_4b86_9699_47c6f7aecd06
  Action Port : ActionPort  ActionType=else
  CopyRight2 : Subsystem  Description=|  mask(Copyright Information){none=on}
      | Copyright info block.                                               
      |                                                                     
      | Place copyright information at the top of every subsystem in design.
      mask prompts: none "No parameters"
      mask help: Place copyright information at the top of every subsystem in design.
      mask Display:
      | NxtrConf = 'Nexteer Confidential';
      | 
      | sys = bdroot; %handle for the current model ("system")
      | first = get_param(sys,'Created');
      | first = first(end-3:end);  %year is last four digits
      | 
      | last = get_param(sys,'LastModifiedDate');
      | if isempty(last)
      |     last = datestr(now,'yyyy');
      | else
      |     last = last(end-3:end);
      | end
      | 
      | if strcmp(first,last)
      |     fprintf('%s -- Copyright %s Nexteer',NxtrConf,first)
      | else
      |     fprintf('%s -- %s%s- %s Nexteer',NxtrConf,char(169),first,last)
      | end
  Quad_24_Budget : LnrIntrpn/LnrIntrpn_u16_u16VariXu16VariY  RequirementInfo="{'linktype_rmi_doors' '0000bb42 (/E-STEER Core/SubSystem Specifications/Application Functions/SF99/SF103A Motor Reference Model)' '#SF103A_76' 'true' 'REQ:  SF103A_76' '' } %GIDa_81b62142_3b3a_4640_b29b_a8cb72d358a9"  XTbl=MotRefMdlQuad24VltgSdlX  YTbl=MotRefMdlQuad24VltgSdlY
      settings: AttributesFormatString=Lnr ( u16VariX , u16VariY )
  VltgSdl : Outport  RequirementInfo={} %GIDa_f7a81aa4_40db_4a10_9ec9_25a7fe867d86
  wires:
  AbsMotVelFild/1 -> Quad_24_Budget/1
  Quad_24_Budget/1 -> VltgSdl/1

== system SF103A_MotRefMdl/MotRefMdl/MotRefMdlPer1/CalcMinimumMotorCurrent/F_CalcIqCmd_2/CopyRight2 ==

== system SF103A_MotRefMdl/MotRefMdl/MotRefMdlPer1/CalcMinimumMotorCurrent/WhileIteratorSubsystem/CopyRight2 ==

== system SF103A_MotRefMdl/MotRefMdl/MotRefMdlPer1/CalcMinimumMotorCurrent/WhileIteratorSubsystem/F_CalcIqCmd_3 ==
  InterCalcns : Inport
  MotTqCmd : Inport  Port=2
  "CurrDaxRef " : Inport  Port=3
  Add : Sum
  Bus Selector : BusSelector  OutputSignals=Ke_VoltPerRadPerSec,RelncTqCoeff_Henry_f32
  Product : Product  RndMeth=Zero
  Product1 : Product  Inputs=*/  RndMeth=Zero
  IqRef_Amp : Outport
  wires:
  Bus Selector/2 -> Product/1  "<RelncTqCoeff_Henry_f32>"
  "CurrDaxRef "/1 -> Product/2
  Bus Selector/1 -> Add/1  "<Ke_VoltPerRadPerSec>"
  Product/1 -> Add/2
  Add/1 -> Product1/2
  MotTqCmd/1 -> Product1/1
  Product1/1 -> IqRef_Amp/1
  InterCalcns/1 -> Bus Selector/1

== system SF103A_MotRefMdl/MotRefMdl/MotRefMdlPer1/CalcMinimumMotorCurrent/WhileIteratorSubsystem/F_ImVSIdq_3 ==
  IqRef_Amp : Inport
  IdRef_Amp : Inport  Port=2
  Math Function : Math  Operator=square  SaturateOnIntegerOverflow=on
  Math Function1 : Math  Operator=square  SaturateOnIntegerOverflow=on
  Sum : Sum  Inputs=|++
  ImRefSq_AmpSq : Outport
  wires:
  IqRef_Amp/1 -> Math Function/1
  IdRef_Amp/1 -> Math Function1/1
  Math Function/1 -> Sum/1
  Math Function1/1 -> Sum/2
  Sum/1 -> ImRefSq_AmpSq/1

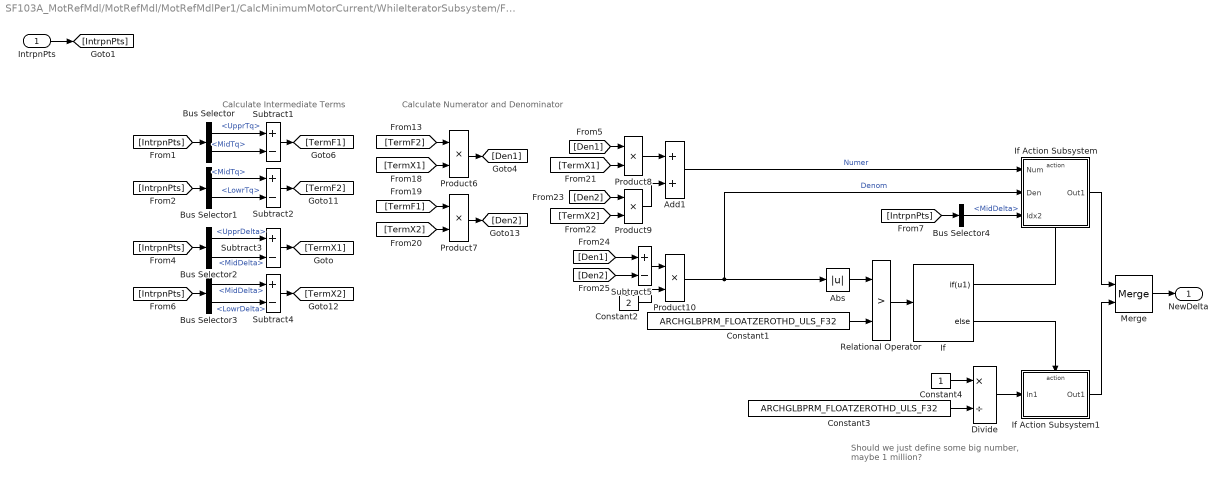
== system SF103A_MotRefMdl/MotRefMdl/MotRefMdlPer1/CalcMinimumMotorCurrent/WhileIteratorSubsystem/F_ParabolicInterpolation ==
  note: Should we just define some big number,
      | maybe 1 million?
  note: Calculate Numerator and Denominator
  note: Calculate Intermediate Terms
  IntrpnPts : Inport
  Abs : Abs
  Add1 : Sum
  Bus Selector : BusSelector  OutputSignals=UpprTq,MidTq
  Bus Selector1 : BusSelector  OutputSignals=MidTq,LowrTq
  Bus Selector2 : BusSelector  OutputSignals=UpprDelta,MidDelta
  Bus Selector3 : BusSelector  OutputSignals=MidDelta,LowrDelta
  Bus Selector4 : BusSelector  OutputSignals=MidDelta
  Constant1 : Constant  Value=ARCHGLBPRM_FLOATZEROTHD_ULS_F32  OutDataTypeStr=single
  Constant2 : Constant  Value=2  OutDataTypeStr=single
  Constant3 : Constant  Value=ARCHGLBPRM_FLOATZEROTHD_ULS_F32  OutDataTypeStr=single
  Constant4 : Constant  OutDataTypeStr=single
  Divide : Product  Inputs=*/
  If : If  IfExpression=u1
  If Action Subsystem : Subsystem  TreatAsAtomicUnit=on
  If Action Subsystem1 : Subsystem  TreatAsAtomicUnit=on
  Merge : Merge
  Product{6..10} (5 alike) : Product
  Relational Operator : RelationalOperator  Operator=>  OutDataTypeStr=boolean
  Subtract{1..5} (5 alike) : Sum  Inputs=+-
  NewDelta : Outport
  wires:
  Subtract1/1 -> [TermF1]
  Subtract2/1 -> [TermF2]
  Subtract3/1 -> [TermX1]
  Subtract4/1 -> [TermX2]
  [TermF2] -> Product6/1
  [TermX1] -> Product6/2
  Product6/1 -> [Den1]
  [TermF1] -> Product7/1
  [TermX2] -> Product7/2
  Product7/1 -> [Den2]
  [Den1] -> Product8/1
  [TermX1] -> Product8/2
  [Den2] -> Product9/1
  [TermX2] -> Product9/2
  Product8/1 -> Add1/1
  Product9/1 -> Add1/2
  Add1/1 -> If Action Subsystem/1(Num)  "Numer"
  [Den1] -> Subtract5/1
  [Den2] -> Subtract5/2
  Subtract5/1 -> Product10/1
  Constant2/1 -> Product10/2
  Product10/1 -> Abs/1, If Action Subsystem/2(Den)  "Denom"
  Constant1/1 -> Relational Operator/2
  Abs/1 -> Relational Operator/1
  Relational Operator/1 -> If/1
  If/1 -> If Action Subsystem/Action
  Constant3/1 -> Divide/2
  Constant4/1 -> Divide/1
  Divide/1 -> If Action Subsystem1/1(In1)
  If/2 -> If Action Subsystem1/Action
  Merge/1 -> NewDelta/1
  If Action Subsystem/1(Out1) -> Merge/1
  If Action Subsystem1/1(Out1) -> Merge/2
  [IntrpnPts] -> Bus Selector/1
  IntrpnPts/1 -> [IntrpnPts]
  Bus Selector/1 -> Subtract1/1  "<UpprTq>"
  Bus Selector/2 -> Subtract1/2  "<MidTq>"
  [IntrpnPts] -> Bus Selector1/1
  Bus Selector1/1 -> Subtract2/1  "<MidTq>"
  Bus Selector1/2 -> Subtract2/2  "<LowrTq>"
  [IntrpnPts] -> Bus Selector2/1
  Bus Selector2/1 -> Subtract3/1  "<UpprDelta>"
  Bus Selector2/2 -> Subtract3/2  "<MidDelta>"
  [IntrpnPts] -> Bus Selector3/1
  Bus Selector3/1 -> Subtract4/1  "<MidDelta>"
  Bus Selector3/2 -> Subtract4/2  "<LowrDelta>"
  [IntrpnPts] -> Bus Selector4/1
  Bus Selector4/1 -> If Action Subsystem/3(Idx2)  "<MidDelta>"

== system SF103A_MotRefMdl/MotRefMdl/MotRefMdlPer1/CalcMinimumMotorCurrent/WhileIteratorSubsystem/Initialize_Points ==
  In1 : Inport
  Action Port : ActionPort  ActionType=then
  Signal Conversion : SignalConversion
  Out1 : Outport
  wires:
  In1/1 -> Signal Conversion/1
  Signal Conversion/1 -> Out1/1

== system SF103A_MotRefMdl/MotRefMdl/MotRefMdlPer1/CalcMinimumMotorCurrent/WhileIteratorSubsystem/Refine_Higher ==
  OldPts : Inport
  NewDelta : Inport  Port=2
  NewTq : Inport  Port=3
  Action Port : ActionPort  ActionType=then
  Bus Creator : BusCreator  Inputs=6
  Bus Selector : BusSelector  OutputSignals=UpprDelta,UpprTq,MidDelta,MidTq
  CopyRight2 : Subsystem  Description=|  mask(Copyright Information){none=on}
      | Copyright info block.                                               
      |                                                                     
      | Place copyright information at the top of every subsystem in design.
      mask prompts: none "No parameters"
      mask help: Place copyright information at the top of every subsystem in design.
      mask Display:
      | NxtrConf = 'Nexteer Confidential';
      | 
      | sys = bdroot; %handle for the current model ("system")
      | first = get_param(sys,'Created');
      | first = first(end-3:end);  %year is last four digits
      | 
      | last = get_param(sys,'LastModifiedDate');
      | if isempty(last)
      |     last = datestr(now,'yyyy');
      | else
      |     last = last(end-3:end);
      | end
      | 
      | if strcmp(first,last)
      |     fprintf('%s -- Copyright %s Nexteer',NxtrConf,first)
      | else
      |     fprintf('%s -- %s%s- %s Nexteer',NxtrConf,char(169),first,last)
      | end
  Data Type Conversion : DataTypeConversion
  Data Type Conversion1 : DataTypeConversion
  Signal Conversion : SignalConversion
  Out1 : Outport
  wires:
  Bus Selector/1 -> Bus Creator/1  "<UpprDelta>"
  Bus Selector/2 -> Bus Creator/2  "<UpprTq>"
  Data Type Conversion/1 -> Bus Creator/5  "LowrDelta"
  Data Type Conversion1/1 -> Bus Creator/6  "LowrTq"
  NewDelta/1 -> Bus Creator/3  "MidDelta"
  NewTq/1 -> Bus Creator/4  "MidTq"
  Bus Creator/1 -> Signal Conversion/1
  OldPts/1 -> Bus Selector/1
  Signal Conversion/1 -> Out1/1
  Bus Selector/3 -> Data Type Conversion/1  "<MidDelta>"
  Bus Selector/4 -> Data Type Conversion1/1  "<MidTq>"

== system SF103A_MotRefMdl/MotRefMdl/MotRefMdlPer1/CalcMinimumMotorCurrent/WhileIteratorSubsystem/Refine_Lower ==
  OldPts : Inport
  NewDelta : Inport  Port=2
  NewTq : Inport  Port=3
  Action Port : ActionPort  ActionType=else
  Bus Creator : BusCreator  Inputs=6
  Bus Selector : BusSelector  OutputSignals=MidDelta,MidTq,LowrDelta,LowrTq
  CopyRight2 : Subsystem  Description=|  mask(Copyright Information){none=on}
      | Copyright info block.                                               
      |                                                                     
      | Place copyright information at the top of every subsystem in design.
      mask prompts: none "No parameters"
      mask help: Place copyright information at the top of every subsystem in design.
      mask Display:
      | NxtrConf = 'Nexteer Confidential';
      | 
      | sys = bdroot; %handle for the current model ("system")
      | first = get_param(sys,'Created');
      | first = first(end-3:end);  %year is last four digits
      | 
      | last = get_param(sys,'LastModifiedDate');
      | if isempty(last)
      |     last = datestr(now,'yyyy');
      | else
      |     last = last(end-3:end);
      | end
      | 
      | if strcmp(first,last)
      |     fprintf('%s -- Copyright %s Nexteer',NxtrConf,first)
      | else
      |     fprintf('%s -- %s%s- %s Nexteer',NxtrConf,char(169),first,last)
      | end
  Data Type Conversion : DataTypeConversion
  Data Type Conversion1 : DataTypeConversion
  Signal Conversion : SignalConversion
  Out1 : Outport
  wires:
  Bus Selector/1 -> Data Type Conversion/1  "<MidDelta>"
  Bus Selector/2 -> Data Type Conversion1/1  "<MidTq>"
  NewDelta/1 -> Bus Creator/3  "MidDelta"
  NewTq/1 -> Bus Creator/4  "MidTq"
  Bus Creator/1 -> Signal Conversion/1
  OldPts/1 -> Bus Selector/1
  Data Type Conversion/1 -> Bus Creator/1  "UpprDelta"
  Data Type Conversion1/1 -> Bus Creator/2  "UpprTq"
  Bus Selector/3 -> Bus Creator/5  "<LowrDelta>"
  Bus Selector/4 -> Bus Creator/6  "<LowrTq>"
  Signal Conversion/1 -> Out1/1

== system SF103A_MotRefMdl/MotRefMdl/MotRefMdlPer1/CalcMinimumMotorCurrent/WhileIteratorSubsystem/Use_Refined_Points ==
  In1 : Inport
  Action Port : ActionPort  ActionType=else
  Signal Conversion : SignalConversion
  Out1 : Outport
  wires:
  In1/1 -> Signal Conversion/1
  Signal Conversion/1 -> Out1/1

== system SF103A_MotRefMdl/MotRefMdl/MotRefMdlPer1/DAxisCurrentBoost/If Action Subsystem/CopyRight2 ==

== system SF103A_MotRefMdl/MotRefMdl/MotRefMdlPer1/DAxisCurrentBoost/If Action Subsystem/CurrToVoltTest  ==
  IdRef_Amp : Inport  RequirementInfo={} %GIDa_f1f46d55_b174_4544_8ce2_404a8ebeeb24
  IqRef_Amp : Inport  RequirementInfo={} %GIDa_c26a37c2_aac9_4e08_9ee9_1ca44c786e0b  Port=2
  InterCalcns : Inport  RequirementInfo={} %GIDa_291c0831_b314_45d6_87ec_0899f7844a1e  Port=3
  Add : Sum  RequirementInfo="{'linktype_rmi_doors' '0000bb42 (/E-STEER Core/SubSystem Specifications/Application Functions/SF99/SF103A Motor Reference Model)' '#SF103A_141' 'true' 'REQ:  SF103A_141' '' } %GIDa_9e50fd45_3b91_4819_a420_04917947868d"  Inputs=+++
  Bus Selector1 : BusSelector  RequirementInfo={} %GIDa_64423790_0274_42ab_8e3c_a1a686db5273  OutputSignals=ReacncQaxOverR,ReacncDaxOverR,EgOverR_Ampr
  Product : Product  RequirementInfo="{'linktype_rmi_doors' '0000bb42 (/E-STEER Core/SubSystem Specifications/Application Functions/SF99/SF103A Motor Reference Model)' '#SF103A_141' 'true' 'REQ:  SF103A_141' '' } %GIDa_80fb7b42_5e1f_4e45_a797_ab2bc89c6f97"  RndMeth=Zero
  Product1 : Product  RequirementInfo="{'linktype_rmi_doors' '0000bb42 (/E-STEER Core/SubSystem Specifications/Application Functions/SF99/SF103A Motor Reference Model)' '#SF103A_141' 'true' 'REQ:  SF103A_141' '' } %GIDa_e9529a08_e424_469d_99e0_5aa2f309e661"  RndMeth=Zero
  Subtract : Sum  RequirementInfo="{'linktype_rmi_doors' '0000bb42 (/E-STEER Core/SubSystem Specifications/Application Functions/SF99/SF103A Motor Reference Model)' '#SF103A_141' 'true' 'REQ:  SF103A_141' '' } %GIDa_8548ced3_d08b_4a2a_82ac_323d0eb9ead4"  Inputs=+-
  VdR_Amp : Outport  RequirementInfo={} %GIDa_a6e4da9b_e4ba_458e_b283_2114740c299f
  VqR_Amp : Outport  RequirementInfo={} %GIDa_1032df96_4a9f_41d8_aa2f_acaa9eb141d7  Port=2
  wires:
  IqRef_Amp/1 -> Add/1, Product/1
  IdRef_Amp/1 -> Subtract/2, Product1/1
  InterCalcns/1 -> Bus Selector1/1
  Bus Selector1/1 -> Product/2  "<ReacncQaxOverR>"
  Bus Selector1/2 -> Product1/2  "<ReacncDaxOverR>"
  Bus Selector1/3 -> Add/3  "<EgOverR_Ampr>"
  Product/1 -> Subtract/1
  Subtract/1 -> VdR_Amp/1
  Product1/1 -> Add/2
  Add/1 -> VqR_Amp/1
